simulink library "TCC_Control_Library"  (R2025b)
settings: Solver=VariableStepAuto  StartTime=0.0  StopTime=10.0  RelTol=1e-3

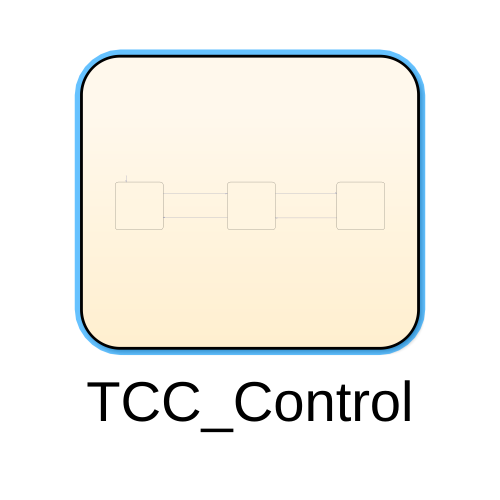
[thumbnail: Simulink's stored preview of the top-level diagram]
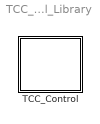
== system TCC_Control_Library ==
  TCC_Control : Stateflow chart  TreatAsAtomicUnit=on

== stateflow chart TCC_Control_Library/TCC_Control ==
  state Release
    during:
    TCC_Control_Solenoid = 0;
  state SlipMode
  state Applied
  (default) -> Release
  SlipMode -> Applied [order 2]
  Release -> SlipMode
  SlipMode -> Release [order 1]
  Applied -> SlipMode
